simulink model "ss11"  (R2021b)
settings: Solver=ode23tb  StartTime=0.0  StopTime=25  FixedStep=1e-06  RelTol=1e-3  EnableMultiTasking=on
undefined symbols (not defined in the file): DiscIntNeverNeededParam, Par, sigbuilder_block, Ts
libraries: fl_lib x36, nesl_utility x30, ee_lib x12, simulink x9, simulink_extras x1, slpidlib x1
(part 1 of 2)
settings Model: SimulationMode=accelerator  Creator=Christo  LastModifiedBy=19840918
settings SolverCC: AlgebraicLoopSolver=TrustRegion  SolverResetMethod=Robust  AutoInsertRateTranBlk=on
settings DataIOCC: LimitDataPoints=on  SaveFormat=Array  ReturnWorkspaceOutputs=off
settings OptimizationCC: LifeSpan=inf
settings DebuggingCC: SolverPrmCheckMsg=warning  SFUnexpectedBacktrackingDiag=warning  SFNoUnconditionalDefaultTransitionDiag=warning  SFExecutionAtInitializationDiag=none  SFMachineParentedDataDiag=warning  ArithmeticOperatorsInVariantConditions=warning
settings HardwareCC: ProdBitPerPointer=32  ProdBitPerSizeT=32  ProdBitPerPtrDiffT=32  ProdLargestAtomicFloat=None  ProdIntDivRoundTo=Undefined  ProdEndianess=Unspecified  ProdWordSize=32  ProdHWDeviceType=32-bit Generic
settings ModelReferenceCC: PropagateSignalLabelsOutOfModel=off
settings SFSimCC: SimUseLocalCustomCode=off  CustomCodeUndefinedFunction=UseInterfaceOnly
settings RTWCC: RTWUseLocalCustomCode=off
settings CodeAppCC: StateflowObjectComments=on
settings GRTTargetCC: TargetLangStandard=C89/C90 (ANSI)
settings ConfigComp: CovMetricSettings=dw  CovSaveCumulativeToWorkspaceVar=on  CovSaveSingleToWorkspaceVar=on  CovExternalEMLEnable=off  CovSFcnEnable=off
settings SimscapeCC: SimscapeNormalizeSystem=off  SimscapeLogOpenViewer=on  SimscapeLogLimitData=off

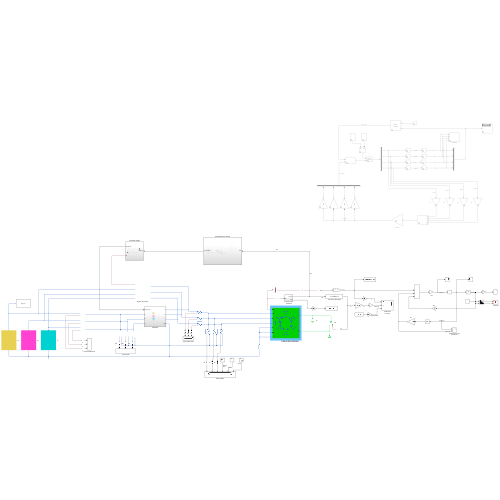
[thumbnail: Simulink's stored preview of the top-level diagram]
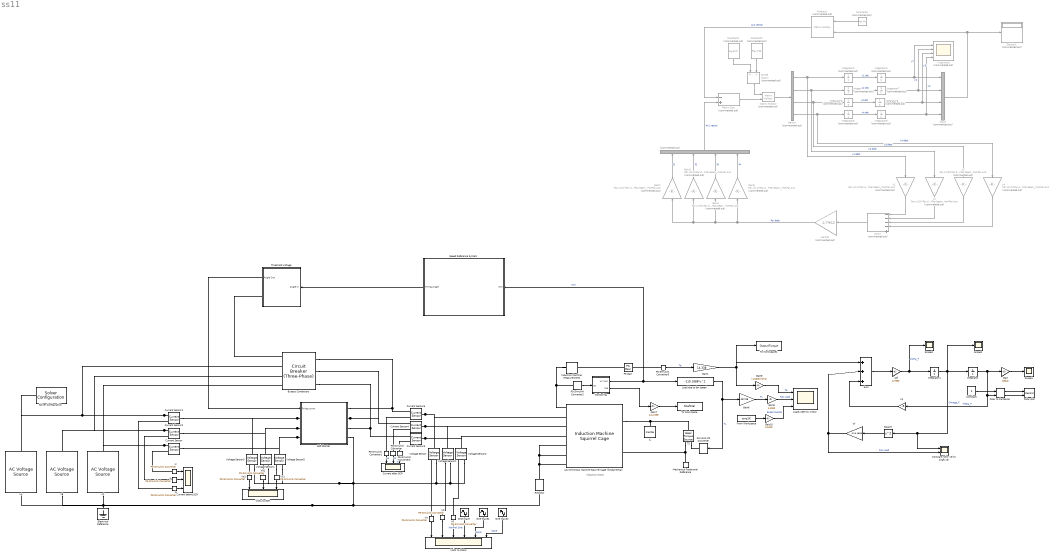
== system ss11 ==
  note: Induction Motor
  . : Mux  Commented=on
  1/Jf : Gain  Gain=1/7962
  Asynchronous Machine Squirrel Cage (fundamental) : ee_lib/Electromechanical/Asynchronous/Induction Machine Squirrel Cage  port_option=ee.enum.threePhasePort.expanded  SRated=250 kW  VRated=690 V  FRated=50 Hz  nPolePairs=2  param_unit=ee.enum.unit.si  squirrel_cage=ee.enum.squirrelcage.Single  zero_sequence=ee.enum.park.zerosequence.include  initialization_option=ee.enum.asm.initialization.fluxvariables  Rs=0.4 Ohm  Xls=0.5 Ohm  pu_Rs=0.0258  pu_Lls=0.0930  Rrd=0.04 Ohm  Xlrd=0.41/6 Ohm  pu_Rrd=0.0145  pu_Llrd=0.0424  Rrd1=0.28 Ohm  Xlrd1=0.82 Ohm  Rrd2=0.28 Ohm  Xlrd2=0.82 Ohm  pu_Rrd1=0.0290  pu_Llrd1=0.0848  pu_Rrd2=0.0290  pu_Llrd2=0.0848  Xm=17 Ohm  pu_Lm=1.7562  X0=0.9 Ohm  pu_L0=0.0930  saturation_option=ee.enum.saturation.exclude  saturation_i=[ 0,4,9,18,25,34,50,68,95,120 ] A  saturation_v=[ 0,88,154,198,220,242,264,286,308,330 ] V  pu_saturation_i=[0, .176, .396, .792, 1.1, 1.496, 2.2, 2.992, 4.18, 5.28]  pu_saturation_v=[0, .2309, .4041, .5196, .5774, .6351, .6928, .7506, .8083, .866]  connection_option=ee.enum.Connection.delta1  angular_position_specify=on  angular_position_priority=High  angular_position=0 deg  angular_position_nominal_specify=off  angular_position_nominal_unit=deg  angular_position_nominal_value=1  pu_psids_specify=off  pu_psids_priority=None  pu_psids=0  pu_psids_nominal_specify=off  pu_psids_nominal_unit=1  pu_psids_nominal_value=1  pu_psiqs_specify=off  pu_psiqs_priority=None  pu_psiqs=0  pu_psiqs_nominal_specify=off  pu_psiqs_nominal_unit=1  pu_psiqs_nominal_value=1  pu_psi0s_specify=off  pu_psi0s_priority=None  pu_psi0s=0  pu_psi0s_nominal_specify=off  pu_psi0s_nominal_unit=1  pu_psi0s_nominal_value=1  pu_psidr_specify=off  pu_psidr_priority=None  pu_psidr=0  pu_psidr_nominal_specify=off  pu_psidr_nominal_unit=1  pu_psidr_nominal_value=1  pu_psiqr_specify=off  pu_psiqr_priority=None  pu_psiqr=0  pu_psiqr_nominal_specify=off  pu_psiqr_nominal_unit=1  pu_psiqr_nominal_value=1  pu_psidr1_specify=off  pu_psidr1_priority=None  pu_psidr1=0  pu_psidr1_nominal_specify=off  pu_psidr1_nominal_unit=1  pu_psidr1_nominal_value=1  pu_psiqr1_specify=off  pu_psiqr1_priority=None  pu_psiqr1=0  pu_psiqr1_nominal_specify=off  pu_psiqr1_nominal_unit=1  pu_psiqr1_nominal_value=1  pu_psidr2_specify=off  pu_psidr2_priority=None  pu_psidr2=0  pu_psidr2_nominal_specify=off  pu_psidr2_nominal_unit=1  pu_psidr2_nominal_value=1  pu_psiqr2_specify=off  pu_psiqr2_priority=None  pu_psiqr2=0  pu_psiqr2_nominal_specify=off  pu_psiqr2_nominal_unit=1  pu_psiqr2_nominal_value=1  psids_specify=off  psids_priority=None  psids=0 Wb  psids_nominal_specify=off  psids_nominal_unit=Wb  psids_nominal_value=1  psiqs_specify=off  psiqs_priority=None  psiqs=0 Wb  psiqs_nominal_specify=off  psiqs_nominal_unit=Wb  psiqs_nominal_value=1  psi0s_specify=off  psi0s_priority=None  psi0s=0 Wb  psi0s_nominal_specify=off  psi0s_nominal_unit=Wb  psi0s_nominal_value=1  psidr_specify=off  psidr_priority=None  psidr=0 Wb  psidr_nominal_specify=off  psidr_nominal_unit=Wb  psidr_nominal_value=1  psiqr_specify=off  psiqr_priority=None  psiqr=0 Wb  psiqr_nominal_specify=off  psiqr_nominal_unit=Wb  psiqr_nominal_value=1  psidr1_specify=off  psidr1_priority=None  psidr1=0 Wb  psidr1_nominal_specify=off  psidr1_nominal_unit=Wb  psidr1_nominal_value=1  psiqr1_specify=off  psiqr1_priority=None  psiqr1=0 Wb  psiqr1_nominal_specify=off  psiqr1_nominal_unit=Wb  psiqr1_nominal_value=1  psidr2_specify=off  psidr2_priority=None  psidr2=0 Wb  psidr2_nominal_specify=off  psidr2_nominal_unit=Wb  psidr2_nominal_value=1  psiqr2_specify=off  psiqr2_priority=None  psiqr2=0 Wb  psiqr2_nominal_specify=off  psiqr2_nominal_unit=Wb  psiqr2_nominal_value=1  slip_specify=off  slip_priority=None  slip=0  slip_nominal_specify=off  slip_nominal_unit=1  slip_nominal_value=1  real_power_generated_specify=off  real_power_generated_priority=None  real_power_generated=0 W  real_power_generated_nominal_specify=off  real_power_generated_nominal_unit=W  real_power_generated_nominal_value=1  mechanical_power_consumed_specify=off  mechanical_power_consumed_priority=None  mechanical_power_consumed=0 W  mechanical_power_consumed_nominal_specify=off  mechanical_power_consumed_nominal_unit=W  mechanical_power_consumed_nominal_value=1  Tmeas=298.15 K  alpha=3.93e-3 1/K  alpha_cage=4.4e-3 1/K  stator_thermal_mass=100 J/K  rotor_thermal_mass=200 J/K  temperatureA_specify=off  temperatureA_priority=High  temperatureA=25 degC  temperatureA_nominal_specify=off  temperatureA_nominal_unit=degC  temperatureA_nominal_value=1  temperatureB_specify=off  temperatureB_priority=High  temperatureB=25 degC  temperatureB_nominal_specify=off  temperatureB_nominal_unit=degC  temperatureB_nominal_value=1  temperatureC_specify=off  temperatureC_priority=High  temperatureC=25 degC  temperatureC_nominal_specify=off  temperatureC_nominal_unit=degC  temperatureC_nominal_value=1  temperatureR_specify=off  temperatureR_priority=High  temperatureR=25 degC  temperatureR_nominal_specify=off  temperatureR_nominal_unit=degC  temperatureR_nominal_value=1
      settings: SourceProductBaseCode=PS  InternalSimscapePortConfiguration="{\"Bottom\":[],\"Left\":[{\"id\":\"R\",\"label\":\"R\",\"type\":\"foundation.mechanical.rotational.rotational\"},{\"id\":\"C\",\"label\":\"C\",\"type\":\"foundation.mechanical.rotational.rotational\"}],\"Right\":[{\"id\":\"pu_output\",\"label\":\"pu\",\"type\":\"output\"},{\"id\":\"a1\",\"label\":\"a1\",\"type\":\"foundation.electrical.electrical\"},{\"id\":\"b1\",\"label\":\"b1\",\"type\":\"foundation.electrical.electrical\"},{\"id\":\"c1\",\"label\":\"c1\",\"type\":\"foundation.electrical.electrical\"},{\"id\":\"a2\",\"label\":\"a2\",\"type\":\"foundation.electrical.electrical\"},{\"id\":\"b2\",\"label\":\"b2\",\"type\":\"foundation.electrical.electrical\"},{\"id\":\"c2\",\"label\":\"c2\",\"type\":\"foundation.electrical.electrical\"}],\"Top\":[]}"
  Bypass Contactors : ee_lib/Switches & Breakers/Circuit Breaker (Three-Phase)  R_closed=0.0001 Ohm  G_open=1e-6 1/Ohm  threshold=2 V
      settings: SourceProductBaseCode=PS  LogSimulationData=on  InternalSimscapePortConfiguration="{\"Bottom\":[],\"Left\":[{\"id\":\"vT\",\"label\":\"vT\",\"type\":\"input\"},{\"id\":\"a1\",\"label\":\"a1\",\"type\":\"foundation.electrical.electrical\"},{\"id\":\"b1\",\"label\":\"b1\",\"type\":\"foundation.electrical.electrical\"},{\"id\":\"c1\",\"label\":\"c1\",\"type\":\"foundation.electrical.electrical\"}],\"Right\":[{\"id\":\"a2\",\"label\":\"a2\",\"type\":\"foundation.electrical.electrical\"},{\"id\":\"b2\",\"label\":\"b2\",\"type\":\"foundation.electrical.electrical\"},{\"id\":\"c2\",\"label\":\"c2\",\"type\":\"foundation.electrical.electrical\"}],\"Top\":[]}"
  Compare rotor vel to shaft vel : Scope  NumInputPorts=2
  Constant : Constant
  Constant1 : Constant  Commented=on  Value=eye(4)
  Constant2 : Constant  Commented=on  Value=Par.Mb
  Constant3 : Constant  Commented=on  Value=Par.Kb
  Current Sensor{,1..5} (6 alike) : fl_lib/Electrical/Electrical Sensors/Current Sensor
  Current after SCR : Scope  NumInputPorts=3
  Current before SCR : Scope  NumInputPorts=3
  Demux : Demux  Commented=on
  Display1 : Display  Commented=on
  Divide : Product  Commented=on  Inputs=*/  Multiplication=Matrix(*)
  Electrical Reference : fl_lib/Electrical/Electrical Elements/Electrical Reference
  From Workspace : FromWorkspace  VariableName=torq1K
  Gain : Gain  Gain=180/pi
  Gain1 : Gain  Gain=14.338
  Gain10 : Gain  Gain=1/1000
  Gain2 : Gain  Commented=on  Gain=Par.xc(1)*Par.delta_x*Par.beam_rho*Par.Acs
  Gain3 : Gain  Commented=on  Gain=Par.xc(2)*Par.delta_x*Par.beam_rho*Par.Acs
  Gain4 : Gain  Commented=on  Gain=Par.xc(3)*Par.delta_x*Par.beam_rho*Par.Acs
  Gain5 : Gain  Commented=on  Gain=Par.xc(4)*Par.delta_x*Par.beam_rho*Par.Acs
  Gain6 : Gain  Gain=-157.08
  Gain7 : Gain  Gain=1/14.338
  Gain8 : Gain  Gain=(1/1000)*2*pi
  Gain9 : Gain  Gain=1/1000
  Ia : nesl_utility/PS-Simulink Converter  PhysicalDomain=network_engine_domain  SubClassName=ps_output  LeftPortType=input  RightPortType=output  PseudoPeriodic=off  Frequencies=[]  Unit=A  AffineConversion=off
      settings: SourceProductBaseCode=PW,SS
  Ib : nesl_utility/PS-Simulink Converter  PhysicalDomain=network_engine_domain  SubClassName=ps_output  LeftPortType=input  RightPortType=output  PseudoPeriodic=off  Frequencies=[]  Unit=A  AffineConversion=off
      settings: SourceProductBaseCode=PW,SS
  Ic : nesl_utility/PS-Simulink Converter  PhysicalDomain=network_engine_domain  SubClassName=ps_output  LeftPortType=input  RightPortType=output  PseudoPeriodic=off  Frequencies=[]  Unit=A  AffineConversion=off
      settings: SourceProductBaseCode=PW,SS
  Induction Machine Measurement1 : ee_lib/Electromechanical/Asynchronous/Induction Machine Measurement  output_idx=1
      settings: SourceProductBaseCode=PS  InternalSimscapePortConfiguration="{\"Bottom\":[],\"Left\":[{\"id\":\"pu_input\",\"label\":\"pu\",\"type\":\"input\"}],\"Right\":[{\"id\":\"pu_output\",\"label\":\"o\",\"type\":\"output\"}],\"Top\":[]}"
  Inertias : Gain  Commented=on  Gain=1/7962
  Integrator : Integrator
  Integrator1 : Integrator
  Integrator{2..9} (8 alike) : Integrator  Commented=on
  JL : fl_lib/Mechanical/Rotational Elements/Inertia  inertia=6.3+10+7962/(14.32^2) kg*m^2  num_ports=foundation.enum.numPorts2.one  w_specify=off  w_priority=High  w=0 rad/s  w_nominal_specify=off  w_nominal_unit=rad/s  w_nominal_value=1  t_specify=off  t_priority=High  t=0 N*m  t_nominal_specify=off  t_nominal_unit=N*m  t_nominal_value=1
  Kf : Gain  Gain=-119.1888
  Ks : Gain  Gain=-5
  Load due to fan speed : Fcn  Expr=-119.1888*u^2
  Loads seen by motor : Scope  NumInputPorts=3
  Matrix Sum : Sum  Commented=on  Inputs=-+
  Matrix Multiply : Product  Commented=on  Multiplication=Matrix(*)
  Mechanical Rotational Reference : fl_lib/Mechanical/Rotational Elements/Mechanical Rotational Reference
  Monitoring : Subsystem
  Mux2 : Mux  Commented=on
  PS Gain : fl_lib/Physical Signals/Functions/PS Gain  gain=1591.55 N*m
  PS-Simulink Converter{,1,3,5} (4 alike) : nesl_utility/PS-Simulink Converter  PhysicalDomain=network_engine_domain  SubClassName=ps_output  LeftPortType=input  RightPortType=output  PseudoPeriodic=off  Frequencies=[]  Unit=inherit  AffineConversion=off
      settings: SourceProductBaseCode=PW,SS
  PS-Simulink Converter2 : nesl_utility/PS-Simulink Converter  PhysicalDomain=network_engine_domain  SubClassName=ps_output  LeftPortType=input  RightPortType=output  PseudoPeriodic=off  Frequencies=[]  Unit=1  AffineConversion=off
      settings: SourceProductBaseCode=PW,SS
  Polar plot : Record  FileSettingsInternal="{\"entries\":[{\"content\":{\"excelSettings\":{\"content\":{},\"type\":\"Streamout.ExcelSettings\"}},\"type\":\"Streamout.FileSettingStorage\",\"uuid\":\"54fc2ee3-5b5e-4f8c-8741-d132ad52efdf\"}],\"packageUris\":[\"http://schema.mathworks.com/mf0/streamout_blocks/R2020a\"],\"version\":\"1.0\"}"  Layout=[1 1]  SignalsInternal="{\"entries\":[{\"content\":{\"signals\":[{\"content\":{\"blockPath\":[\"ss11/Polar plot\"],\"channel\":[],\"dimensions\":[1],\"domain\":\"ss11/Polar plot\",\"lineColor\":\"#77ac30\",\"plots\":[],\"port\":1,\"sid\":[\"\"],\"signalID\":639,\"signalName\":\"Polar to\\nCartesian:1\"},\"type\":\"RecordBlkView.Signal\",\"uuid\":\"d88677cd-d414-4038-8e24-bb5f350f4e87\"},{\"content\":{\"blockPath\":[\"ss11/Polar plot\"],\"channel\":[],\"dimensions\":[1],\"domain\":\"ss11/Polar plot\",\"lineColor\":\"#4dbeee\",\"plots\":[],\"port\":2,\"sid\":[\"\"],\"signalID\":643,\"signalName\":\"Polar to\\nCartesian:2\"},\"type\":\"RecordBlkView.Signal\",\"uuid\":\"c3000e72-a674-483a-a6e8-47c6664286a5\"}]},\"type\":\"RecordBlkView.InputSignals\",\"uuid\":\"32de7f82-7389-4a3b-8503-0a628280bb19\"}],\"packageUris\":[\"http://schema.mathworks.com/mf0/streamout_blocks/R2020a\"],\"version\":\"1.0\"}"  VisualizationBindings="{\"xyplotplugin\":{\"info\":[{\"series\":[],\"subplotID\":1}]}}"  CompatibilityTag=XY
  Polar to Cartesian : simulink_extras/Transformations/Polar to Cartesian
      settings: SourceProductBaseCode=SL
  Product1 : Product  Commented=on  Multiplication=Matrix(*)
  Resistor : fl_lib/Electrical/Electrical Elements/Resistor  R=1e09 Ohm  i_specify=off  i_priority=None  i=0 A  i_nominal_specify=off  i_nominal_unit=A  i_nominal_value=1  v_specify=off  v_priority=None  v=0 V  v_nominal_specify=off  v_nominal_unit=V  v_nominal_value=1
  Scope1 : Scope
  Scope2 : Scope
  Scope3 : Scope
  Simulink-PS Converter : nesl_utility/Simulink-PS Converter  PhysicalDomain=network_engine_domain  SubClassName=ps_input  LeftPortType=input  RightPortType=output  PseudoPeriodic=off  Frequencies=[]  NoiseDistribution=none  NoiseParameters=[]  Unit=N*m  AffineConversion=off  FilteringAndDerivatives=zero  SimscapeFilterOrder=1  InputFilterTimeConstant=0.001  UdotUserProvided=1
      settings: SourceProductBaseCode=PW,SS
  Sine Wave : Sin  Amplitude=690  Frequency=2*pi*50  SampleTime=0
  Sine Wave1 : Sin  Amplitude=690  Frequency=2*pi*50  Phase=2*pi/3  SampleTime=0
  Sine Wave2 : Sin  Amplitude=690  Frequency=2*pi*50  Phase=-2*pi/3  SampleTime=0
  Soft Starter : Subsystem
  Solver Configuration : nesl_utility/Solver Configuration  PhysicalDomain=network_engine_domain  SubClassName=solver  LeftPortType=input  RightPortType=generic  Tones=[]  Harmonics=[]  SimulateNoise=off  Profile=off  UseLocalSampling=off  EnableSwitchedLinearOptims=on  FrequencyDomain=off  UseCCode=off  RelTol=0.001  AbsTol=1e-06  MinStep=1e-09  ToWorkspace=off  RevertToSquareIcSolve=off  NumHomotopyIterations=100  PhasorMode=off  PhasorModeNumHarmonics=1  DoDC=off  ResidualTolerance=1e-09  UseLocalSolver=on  LocalSolverChoice=NE_BACKWARD_EULER_ADVANCER  LocalSolverSampleTime=1.0e-04  DoFixedCost=on  MaxNonlinIter=3  MaxModeIter=2  ComputeImpulses=off  ImpulseIterations=2  LinearAlgebra=Sparse  EquationFormulation=NE_TIME_EF  DelaysMemoryBudget=1024  AutomaticFiltering=on  FilteringTimeConstant=0.001  PartitionStorageMethod=AS_NEEDED  PartitionMemoryBudget=1024  PartitionMethod=FAST
      settings: SourceProductBaseCode=PW,SS
  Speed Reference System : Subsystem
  Square : Math  Operator=square  SaturateOnIntegerOverflow=on
  Sum : Sum  Inputs=|+++
  Sum2 : Sum  Commented=on  Inputs=----+
  TS : fl_lib/Mechanical/Mechanical Sources/Ideal Torque Source
  Threshold Voltage : Subsystem
  To Workspace : ToWorkspace  VariableName=ShaftVel  SaveFormat=Timeseries  SampleTime=-1
  To Workspace1 : ToWorkspace  VariableName=OutputTorque  SaveFormat=Timeseries  SampleTime=-1
  Va : nesl_utility/PS-Simulink Converter  PhysicalDomain=network_engine_domain  SubClassName=ps_output  LeftPortType=input  RightPortType=output  PseudoPeriodic=off  Frequencies=[]  Unit=inherit  AffineConversion=off
      settings: SourceProductBaseCode=PW,SS
  Va1 : nesl_utility/PS-Simulink Converter  PhysicalDomain=network_engine_domain  SubClassName=ps_output  LeftPortType=input  RightPortType=output  PseudoPeriodic=off  Frequencies=[]  Unit=inherit  AffineConversion=off
      settings: SourceProductBaseCode=PW,SS
  Vb : nesl_utility/PS-Simulink Converter  PhysicalDomain=network_engine_domain  SubClassName=ps_output  LeftPortType=input  RightPortType=output  PseudoPeriodic=off  Frequencies=[]  Unit=inherit  AffineConversion=off
      settings: SourceProductBaseCode=PW,SS
  Vb1 : nesl_utility/PS-Simulink Converter  PhysicalDomain=network_engine_domain  SubClassName=ps_output  LeftPortType=input  RightPortType=output  PseudoPeriodic=off  Frequencies=[]  Unit=inherit  AffineConversion=off
      settings: SourceProductBaseCode=PW,SS
  Vc : nesl_utility/PS-Simulink Converter  PhysicalDomain=network_engine_domain  SubClassName=ps_output  LeftPortType=input  RightPortType=output  PseudoPeriodic=off  Frequencies=[]  Unit=inherit  AffineConversion=off
      settings: SourceProductBaseCode=PW,SS
  Vc1 : nesl_utility/PS-Simulink Converter  PhysicalDomain=network_engine_domain  SubClassName=ps_output  LeftPortType=input  RightPortType=output  PseudoPeriodic=off  Frequencies=[]  Unit=inherit  AffineConversion=off
      settings: SourceProductBaseCode=PW,SS
  Voltage Sensor{,1..5} (6 alike) : fl_lib/Electrical/Electrical Sensors/Voltage Sensor
  Volts to Motor : Scope  NumInputPorts=6
  Volts to SCR : Scope  NumInputPorts=3
  Y-positions : Scope  Commented=on  NumInputPorts=4
  vA : fl_lib/Electrical/Electrical Sources/AC Voltage Source  amp=690 V  shift=0 deg  frequency=50 Hz  omega=0 rad/s
  vB : fl_lib/Electrical/Electrical Sources/AC Voltage Source  amp=690 V  shift=-120 deg  frequency=50 Hz  omega=0 rad/s
  vC : fl_lib/Electrical/Electrical Sources/AC Voltage Source  amp=690 V  shift=120 deg  frequency=50 Hz  omega=0 rad/s
  y1 : Gain  Commented=on  Gain=Par.xc(1)*Par.delta_x*Par.beam_rho*Par.Acs
  y2 : Gain  Commented=on  Gain=Par.xc(2)*Par.delta_x*Par.beam_rho*Par.Acs
  y3 : Gain  Commented=on  Gain=Par.xc(3)*Par.delta_x*Par.beam_rho*Par.Acs
  y4 : Gain  Commented=on  Gain=Par.xc(4)*Par.delta_x*Par.beam_rho*Par.Acs
  wires:
  PS-Simulink Converter2/1 -> Monitoring/1(pu)
  PS-Simulink Converter5/1 -> Gain1/1  "Te"
  Vb/1 -> Volts to Motor/2
  PS-Simulink Converter1/1 -> Current after SCR/1  "Ia"
  PS-Simulink Converter3/1 -> Current after SCR/3  "Ic"
  PS-Simulink Converter/1 -> Current after SCR/2  "Ib"
  Ia/1 -> Current before SCR/3
  Ib/1 -> Current before SCR/2
  1/Jf/1 -> Integrator1/1, Scope3/1  "Alpha_F"
  Gain/1 -> Scope1/1
  Polar to Cartesian/2 -> Polar plot/2
  Constant/1 -> Polar to Cartesian/1
  Polar to Cartesian/1 -> Polar plot/1
  Speed Reference System/1(Firing Angle) -> Threshold Voltage/1(Angle In)
  Threshold Voltage/1(Angle Out) -> Soft Starter/1(firing curve)
  Monitoring/1(wr (pu)) -> Load due to fan speed/1, Speed Reference System/1(Win)  "Win"
  Ic/1 -> Current before SCR/1
  Sine Wave2/1 -> Volts to Motor/6  "-2pi/3"
  Sine Wave/1 -> Volts to Motor/4  "Normal Sine"
  Integrator/1 -> Gain/1, Ks/1, Polar to Cartesian/2  "Theta_F"
  Va1/1 -> Volts to SCR/1
  Va/1 -> Volts to Motor/1
  Kf/1 -> Compare rotor vel to shaft vel/2, Sum/2  "Fan Load"
  Sine Wave1/1 -> Volts to Motor/5  "2pi/3"
  Square/1 -> Kf/1
  Integrator1/1 -> Integrator/1, Scope2/1, Compare rotor vel to shaft vel/1, Square/1  "Omega_F"
  Vc/1 -> Volts to Motor/3
  Sum/1 -> 1/Jf/1
  Vc1/1 -> Volts to SCR/3
  Vb1/1 -> Volts to SCR/2
  y4/1 -> Sum2/4
  Demux/3 -> Integrator5/1, y3/1  "y3 ddot"
  Gain2/1 -> ./1  "f1"
  Integrator3/1 -> Y-positions/1, Mux2/1  "y1"
  y3/1 -> Sum2/3
  Integrator4/1 -> Integrator7/1  "y2 dot"
  Demux/1 -> Integrator2/1, y1/1  "y1 ddot"
  Integrator9/1 -> Y-positions/4, Mux2/4  "y4"
  Gain3/1 -> ./2  "f2"
  Constant3/1 -> Product1/1
  Integrator8/1 -> Y-positions/3, Mux2/3  "y3"
  Inertias/1 -> Gain2/1, Gain3/1, Gain4/1, Gain5/1  "Psi ddot"
  y1/1 -> Sum2/1
  Matrix Multiply/1 -> Demux/1
  Constant1/1 -> Divide/1
  Integrator5/1 -> Integrator8/1  "y3 dot"
  Gain5/1 -> ./4  "f4"
  Gain4/1 -> ./3  "f3"
  Demux/4 -> Integrator6/1, y4/1  "y4 ddot"
  Integrator7/1 -> Y-positions/2, Mux2/2  "y2"
  Sum2/1 -> Inertias/1
  y2/1 -> Sum2/2
  Demux/2 -> Integrator4/1, y2/1  "y2 ddot"
  Divide/1 -> Matrix Multiply/1
  Product1/1 -> Matrix Sum/1  "4x1 vector"
  Integrator2/1 -> Integrator3/1  "y1 dot"
  Matrix Sum/1 -> Matrix Multiply/2
  Constant2/1 -> Divide/2
  Integrator6/1 -> Integrator9/1  "y4 dot"
  Mux2/1 -> Product1/2, Display1/1
  ./1 -> Matrix Sum/2  "4x1 vector"
  Load due to fan speed/1 -> Simulink-PS Converter/1, Gain6/1  "TL"
  Gain1/1 -> Sum/1, To Workspace1/1, Gain8/1
  Ks/1 -> Sum/3
  Gain7/1 -> To Workspace/1
  Monitoring/2(We) -> Gain7/1
  Gain6/1 -> Gain9/1  "TL"
  Gain9/1 -> Loads seen by motor/2  "Fan Load"
  Gain10/1 -> Loads seen by motor/3  "Experimental"
  From Workspace/1 -> Gain10/1
  Gain8/1 -> Loads seen by motor/1  "Te"
  connections:
  Current Sensor4/LConn1 -- Asynchronous Machine Squirrel Cage (fundamental)/RConn3 -- Voltage Sensor1/LConn1
  Soft Starter/RConn2 -- Current Sensor4/RConn2 -- Bypass Contactors/RConn2
  Current Sensor1/RConn2 -- Bypass Contactors/LConn2 -- vA/LConn1 -- Solver Configuration/RConn1
  Soft Starter/LConn3 -- Current Sensor/LConn1 -- Voltage Sensor5/LConn1
  Current Sensor5/LConn1 -- Asynchronous Machine Squirrel Cage (fundamental)/RConn2 -- Voltage Sensor/LConn1
  TS/RConn2 -- Asynchronous Machine Squirrel Cage (fundamental)/LConn2 -- Mechanical Rotational Reference/LConn1
  Asynchronous Machine Squirrel Cage (fundamental)/RConn7 -- Asynchronous Machine Squirrel Cage (fundamental)/RConn5 -- Asynchronous Machine Squirrel Cage (fundamental)/RConn6 -- Resistor/LConn1
  Soft Starter/LConn2 -- Current Sensor2/LConn1 -- Voltage Sensor4/LConn1
  Bypass Contactors/RConn1 -- Soft Starter/RConn1 -- Current Sensor5/RConn2
  JL/LConn1 -- TS/LConn1 -- Asynchronous Machine Squirrel Cage (fundamental)/LConn1
  Bypass Contactors/RConn3 -- Soft Starter/RConn3 -- Current Sensor3/RConn2
  Current Sensor3/LConn1 -- Asynchronous Machine Squirrel Cage (fundamental)/RConn4 -- Voltage Sensor2/LConn1
  Voltage Sensor2/RConn2 -- Voltage Sensor3/RConn2 -- Voltage Sensor4/RConn2 -- Voltage Sensor5/RConn2 -- Soft Starter/RConn4 -- Resistor/RConn1 -- Electrical Reference/LConn1 -- vC/RConn1 -- vA/RConn1 -- vB/RConn1 -- Voltage Sensor/RConn2 -- Voltage Sensor1/RConn2
  Current Sensor2/RConn2 -- vB/LConn1 -- Bypass Contactors/LConn3
  Induction Machine Measurement1/LConn1 -- PS-Simulink Converter2/LConn1 -- Asynchronous Machine Squirrel Cage (fundamental)/RConn1
  Current Sensor/RConn2 -- vC/LConn1 -- Bypass Contactors/LConn4
  Soft Starter/LConn1 -- Current Sensor1/LConn1 -- Voltage Sensor3/LConn1
  Current Sensor3/RConn1 -- PS-Simulink Converter3/LConn1
  Voltage Sensor4/RConn1 -- Vb1/LConn1
  Current Sensor1/RConn1 -- Ia/LConn1
  Va1/LConn1 -- Voltage Sensor3/RConn1
  PS-Simulink Converter1/LConn1 -- Current Sensor5/RConn1
  PS Gain/LConn1 -- Induction Machine Measurement1/RConn1
  Threshold Voltage/RConn1 -- Bypass Contactors/LConn1
  Va/LConn1 -- Voltage Sensor/RConn1
  Current Sensor4/RConn1 -- PS-Simulink Converter/LConn1
  Vc/LConn1 -- Voltage Sensor2/RConn1
  Voltage Sensor5/RConn1 -- Vc1/LConn1
  Voltage Sensor1/RConn1 -- Vb/LConn1
  Current Sensor2/RConn1 -- Ib/LConn1
  Ic/LConn1 -- Current Sensor/RConn1
  PS-Simulink Converter5/LConn1 -- PS Gain/RConn1
  TS/RConn1 -- Simulink-PS Converter/RConn1

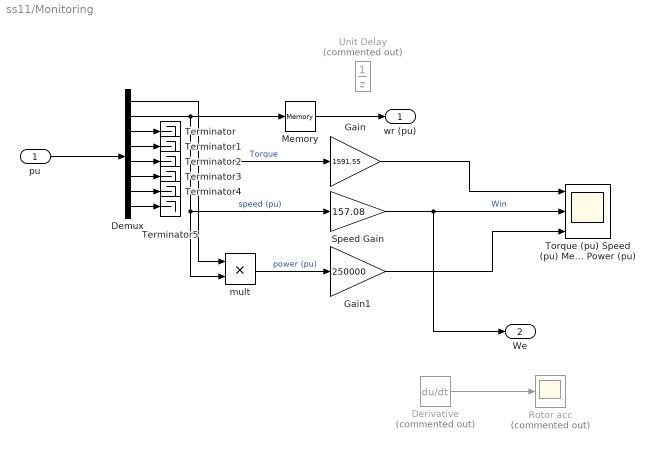
== system ss11/Monitoring ==
  pu : Inport
  Demux : Demux  Outputs=8
  Derivative : Derivative  Commented=on
  Gain : Gain  Gain=1591.55
  Gain1 : Gain  Gain=250000
  Memory : Memory
  Rotor acc : Scope  Commented=on
  Speed Gain : Gain  Gain=157.08
  Terminator{,1..5} (6 alike) : Terminator
  "Torque (pu) Speed (pu) Mech Power (pu) " : Scope  NumInputPorts=3
  Unit Delay : UnitDelay  Commented=on  SampleTime=-1  HasFrameUpgradeWarning=on
  mult : Product  Inputs=**
  wr (pu) : Outport
  We : Outport  Port=2
  wires:
  pu/1 -> Demux/1
  Demux/2 -> Memory/1, mult/2, Speed Gain/1  "speed (pu)"
  mult/1 -> Gain1/1  "power (pu)"
  Demux/1 -> mult/1, Gain/1  "Torque"
  Demux/3 -> Terminator/1
  Demux/8 -> Terminator5/1
  Demux/7 -> Terminator4/1
  Demux/6 -> Terminator3/1
  Demux/5 -> Terminator2/1
  Demux/4 -> Terminator1/1
  Gain1/1 -> "Torque (pu) Speed (pu) Mech Power (pu) "/3
  Derivative/1 -> Rotor acc/1
  Speed Gain/1 -> We/1, "Torque (pu) Speed (pu) Mech Power (pu) "/2  "Win"
  Gain/1 -> "Torque (pu) Speed (pu) Mech Power (pu) "/1
  Memory/1 -> wr (pu)/1

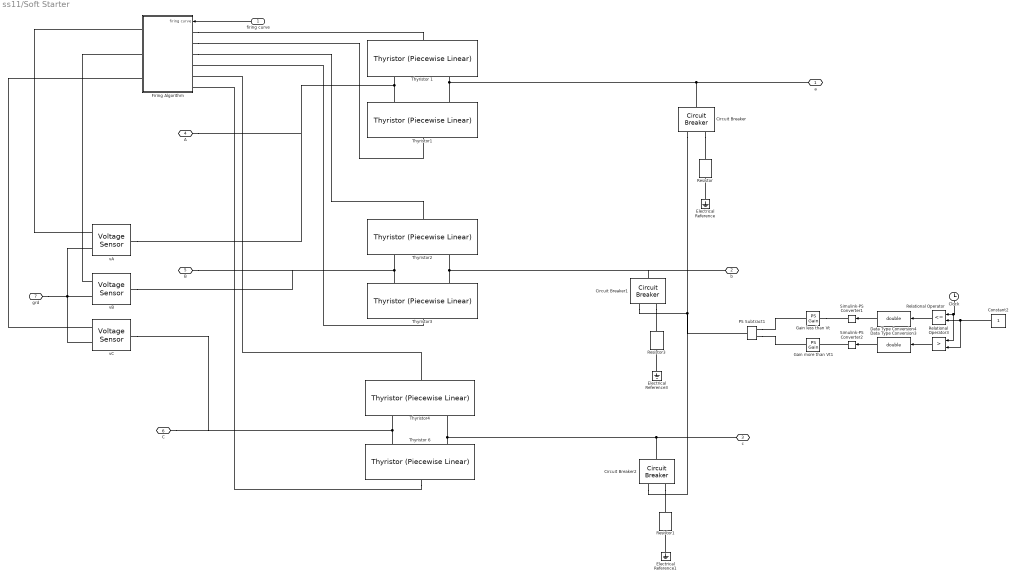
== system ss11/Soft Starter ==
  firing curve : Inport
  Circuit Breaker : ee_lib/Switches & Breakers/Circuit Breaker  R_closed=0.001 Ohm  G_open=1e-6 1/Ohm  threshold=2 V  offset_for_on=1 V
      settings: SourceProductBaseCode=PS  InternalSimscapePortConfiguration="{\"Bottom\":[],\"Left\":[{\"id\":\"vT\",\"label\":\"vT\",\"type\":\"input\"},{\"id\":\"p1\",\"label\":\"\",\"type\":\"foundation.electrical.electrical\"}],\"Right\":[{\"id\":\"p2\",\"label\":\"\",\"type\":\"foundation.electrical.electrical\"}],\"Top\":[]}"
  Circuit Breaker1 : ee_lib/Switches & Breakers/Circuit Breaker  R_closed=0.001 Ohm  G_open=1e-6 1/Ohm  threshold=2 V  offset_for_on=1 V
      settings: SourceProductBaseCode=PS  InternalSimscapePortConfiguration="{\"Bottom\":[],\"Left\":[{\"id\":\"vT\",\"label\":\"vT\",\"type\":\"input\"},{\"id\":\"p1\",\"label\":\"\",\"type\":\"foundation.electrical.electrical\"}],\"Right\":[{\"id\":\"p2\",\"label\":\"\",\"type\":\"foundation.electrical.electrical\"}],\"Top\":[]}"
  Circuit Breaker2 : ee_lib/Switches & Breakers/Circuit Breaker  R_closed=0.001 Ohm  G_open=1e-6 1/Ohm  threshold=2 V  offset_for_on=1 V
      settings: SourceProductBaseCode=PS  InternalSimscapePortConfiguration="{\"Bottom\":[],\"Left\":[{\"id\":\"vT\",\"label\":\"vT\",\"type\":\"input\"},{\"id\":\"p1\",\"label\":\"\",\"type\":\"foundation.electrical.electrical\"}],\"Right\":[{\"id\":\"p2\",\"label\":\"\",\"type\":\"foundation.electrical.electrical\"}],\"Top\":[]}"
  Clock : Clock
  Constant2 : Constant
  Data Type Conversion3 : DataTypeConversion  OutDataTypeStr=double
  Data Type Conversion4 : DataTypeConversion  OutDataTypeStr=double
  Electrical Reference : fl_lib/Electrical/Electrical Elements/Electrical Reference
  Electrical Reference1 : fl_lib/Electrical/Electrical Elements/Electrical Reference
  Electrical Reference3 : fl_lib/Electrical/Electrical Elements/Electrical Reference
  Firing Algorithm : Subsystem
  Gain less than Vt : fl_lib/Physical Signals/Functions/PS Gain  gain=-1 V
  Gain more than Vt1 : fl_lib/Physical Signals/Functions/PS Gain  gain=3 V
  PS Subtract1 : fl_lib/Physical Signals/Functions/PS Subtract
  Relational Operator : RelationalOperator  Operator=<=  OutDataTypeStr=boolean  RndMeth=Simplest
  Relational Operator3 : RelationalOperator  Operator=>  OutDataTypeStr=boolean  RndMeth=Simplest
  Resistor : fl_lib/Electrical/Electrical Elements/Resistor  R=0.01 Ohm  i_specify=off  i_priority=None  i=0 A  i_nominal_specify=off  i_nominal_unit=A  i_nominal_value=1  v_specify=off  v_priority=None  v=0 V  v_nominal_specify=off  v_nominal_unit=V  v_nominal_value=1
  Resistor1 : fl_lib/Electrical/Electrical Elements/Resistor  R=0.01 Ohm  i_specify=off  i_priority=None  i=0 A  i_nominal_specify=off  i_nominal_unit=A  i_nominal_value=1  v_specify=off  v_priority=None  v=0 V  v_nominal_specify=off  v_nominal_unit=V  v_nominal_value=1
  Resistor3 : fl_lib/Electrical/Electrical Elements/Resistor  R=0.01 Ohm  i_specify=off  i_priority=None  i=0 A  i_nominal_specify=off  i_nominal_unit=A  i_nominal_value=1  v_specify=off  v_priority=None  v=0 V  v_nominal_specify=off  v_nominal_unit=V  v_nominal_value=1
  Simulink-PS Converter1 : nesl_utility/Simulink-PS Converter  PhysicalDomain=network_engine_domain  SubClassName=ps_input  LeftPortType=input  RightPortType=output  PseudoPeriodic=off  Frequencies=[]  NoiseDistribution=none  NoiseParameters=[]  Unit=1  AffineConversion=off  FilteringAndDerivatives=provide  SimscapeFilterOrder=1  InputFilterTimeConstant=0.001  UdotUserProvided=0
      settings: SourceProductBaseCode=PW,SS
  Simulink-PS Converter2 : nesl_utility/Simulink-PS Converter  PhysicalDomain=network_engine_domain  SubClassName=ps_input  LeftPortType=input  RightPortType=output  PseudoPeriodic=off  Frequencies=[]  NoiseDistribution=none  NoiseParameters=[]  Unit=1  AffineConversion=off  FilteringAndDerivatives=provide  SimscapeFilterOrder=1  InputFilterTimeConstant=0.001  UdotUserProvided=0
      settings: SourceProductBaseCode=PW,SS
  Thyristor 1 : ee_lib/Semiconductors & Converters/Thyristor (Piecewise Linear)  Vf=0.8 V  Ron=0.001 Ohm  Goff=1.0000e-05 1/Ohm  Vgt=6 V  Ih=0.01 A  diode_param=1  diode_Vf=0.8 V  diode_Ron=0.001 Ohm  diode_Goff=1e-5 1/Ohm  diode_C=5e-8 F  diode_iRM=-235 A  diode_iF=300 A  diode_idot=-50 A/us  diode_trr_param=1  diode_trr_factor=3  diode_trr=15 us  diode_Qrr=1.5e+3 s*uA  thermal_loss_option=ee.enum.converters.thermalLossOption.constantvalues  Von_data=[0, .1, .6, .8, 1, 1.3, 1.6, 2, 2.4; 0, .1, .7, 1, 1.2, 1.5, 1.9, 2.4, 2.8] V  Tj=[298.15, 398.15] K  Iout_data=[0, .1, 1, 5, 10, 20, 40, 70, 100] A  Eon_data=[0, .0024, .024, .12, .2, .48, 1.04, 2.16, 3.24; 0, .003, .03, .15, .25, .6, 1.3, 2.7, 4.05] * 1e-3 J  Tj_loss=[298.15, 398.15] K  Iout_data_loss=[0, .1, 1, 5, 10, 20, 40, 70, 100] A  Eon_scalar=22.86e-3 J  Eoff_natural_commutation=10e-3 J  Voff=300 V  Iout_scalar=600 A  onCurrentMeasDelay=1e-4 s  diodeModelType=ee.enum.converters.diodeModelType.pwl  diodeTableType=ee.enum.diode.tableType.IfMat  diode_IfMat=[.07, .12, .19, 1.75, 4.24, 7.32, 11.2; .16, .3, .72, 2.14, 4.02, 6.35, 9.12] A  diode_VfMat=[.9, 1.15, 1.25, 1.5, 1.75, 2.17, 2.6, 2.85; .58, .68, .75, 1.1, 1.38, 1.77, 2.27, 2.7] V  diode_TjVec=[25, 125] degC  diode_VfVec=[.5, .7, .9, 1.3, 1.7, 2.1, 2.5] V  diode_IfVec=[.1, .2, .5, 1, 2, 4, 7, 10] A  thermal_network_parameterization=ee.enum.thermalNetworkTopology.external  Rth=[.08, .5] K/W  Rth_Cauer=[.08, .1, .5] K/W  Rth_Foster=[.08, .14, .22, .16] K/W  thermal_mass_parameterization=ee.enum.thermalNetwork.timeconstant  thermal_mass=[.01, .5] J/K  thermal_mass_Cauer=[.01, .1, .5] J/K  thermal_mass_Foster=[.001, .005, .05, .5] J/K  thermal_time_constant=[.001, .2] s  thermal_time_constant_Cauer=[.001, .1, .2] s  thermal_time_constant_Foster=[7e-05, .0007, .01, .08] s  thermal_mass_initial_temperatures=[25, 25] degC  thermal_mass_initial_temperatures_Cauer=[25, 25, 25] degC  junction_thermal_mass=0.01 J/K  steadyState_Foster=simscape.enum.onoff.on  Tvec_initial_Foster=[25, 25, 25, 25] degC  junction_temperature_specify=off  junction_temperature_priority=None  junction_temperature=25 degC  junction_temperature_nominal_specify=off  junction_temperature_nominal_unit=degC  junction_temperature_nominal_value=1  vT_specify=off  vT_priority=None  vT=0 V  vT_nominal_specify=off  vT_nominal_unit=V  vT_nominal_value=1  Qj_specify=off  Qj_priority=None  Qj=0 W  Qj_nominal_specify=off  Qj_nominal_unit=W  Qj_nominal_value=1
      settings: SourceProductBaseCode=PS  LogSimulationData=on  InternalSimscapePortConfiguration="{\"Bottom\":[],\"Left\":[{\"id\":\"G\",\"label\":\"\",\"type\":\"input\"}],\"Right\":[{\"id\":\"A\",\"label\":\"\",\"type\":\"foundation.electrical.electrical\"},{\"id\":\"K\",\"label\":\"\",\"type\":\"foundation.electrical.electrical\"}],\"Top\":[]}"
  Thyristor 6 : ee_lib/Semiconductors & Converters/Thyristor (Piecewise Linear)  Vf=0.8 V  Ron=0.001 Ohm  Goff=1.0000e-05 1/Ohm  Vgt=6 V  Ih=0.01 A  diode_param=1  diode_Vf=0.8 V  diode_Ron=0.001 Ohm  diode_Goff=1e-5 1/Ohm  diode_C=5e-8 F  diode_iRM=-235 A  diode_iF=300 A  diode_idot=-50 A/us  diode_trr_param=1  diode_trr_factor=3  diode_trr=15 us  diode_Qrr=1.5e+3 s*uA  thermal_loss_option=ee.enum.converters.thermalLossOption.constantvalues  Von_data=[0, .1, .6, .8, 1, 1.3, 1.6, 2, 2.4; 0, .1, .7, 1, 1.2, 1.5, 1.9, 2.4, 2.8] V  Tj=[298.15, 398.15] K  Iout_data=[0, .1, 1, 5, 10, 20, 40, 70, 100] A  Eon_data=[0, .0024, .024, .12, .2, .48, 1.04, 2.16, 3.24; 0, .003, .03, .15, .25, .6, 1.3, 2.7, 4.05] * 1e-3 J  Tj_loss=[298.15, 398.15] K  Iout_data_loss=[0, .1, 1, 5, 10, 20, 40, 70, 100] A  Eon_scalar=22.86e-3 J  Eoff_natural_commutation=10e-3 J  Voff=300 V  Iout_scalar=600 A  onCurrentMeasDelay=1e-4 s  diodeModelType=ee.enum.converters.diodeModelType.pwl  diodeTableType=ee.enum.diode.tableType.IfMat  diode_IfMat=[.07, .12, .19, 1.75, 4.24, 7.32, 11.2; .16, .3, .72, 2.14, 4.02, 6.35, 9.12] A  diode_VfMat=[.9, 1.15, 1.25, 1.5, 1.75, 2.17, 2.6, 2.85; .58, .68, .75, 1.1, 1.38, 1.77, 2.27, 2.7] V  diode_TjVec=[25, 125] degC  diode_VfVec=[.5, .7, .9, 1.3, 1.7, 2.1, 2.5] V  diode_IfVec=[.1, .2, .5, 1, 2, 4, 7, 10] A  thermal_network_parameterization=ee.enum.thermalNetworkTopology.external  Rth=[.08, .5] K/W  Rth_Cauer=[.08, .1, .5] K/W  Rth_Foster=[.08, .14, .22, .16] K/W  thermal_mass_parameterization=ee.enum.thermalNetwork.timeconstant  thermal_mass=[.01, .5] J/K  thermal_mass_Cauer=[.01, .1, .5] J/K  thermal_mass_Foster=[.001, .005, .05, .5] J/K  thermal_time_constant=[.001, .2] s  thermal_time_constant_Cauer=[.001, .1, .2] s  thermal_time_constant_Foster=[7e-05, .0007, .01, .08] s  thermal_mass_initial_temperatures=[25, 25] degC  thermal_mass_initial_temperatures_Cauer=[25, 25, 25] degC  junction_thermal_mass=0.01 J/K  steadyState_Foster=simscape.enum.onoff.on  Tvec_initial_Foster=[25, 25, 25, 25] degC  junction_temperature_specify=off  junction_temperature_priority=None  junction_temperature=25 degC  junction_temperature_nominal_specify=off  junction_temperature_nominal_unit=degC  junction_temperature_nominal_value=1  vT_specify=off  vT_priority=None  vT=0 V  vT_nominal_specify=off  vT_nominal_unit=V  vT_nominal_value=1  Qj_specify=off  Qj_priority=None  Qj=0 W  Qj_nominal_specify=off  Qj_nominal_unit=W  Qj_nominal_value=1
      settings: SourceProductBaseCode=PS  InternalSimscapePortConfiguration="{\"Bottom\":[],\"Left\":[{\"id\":\"G\",\"label\":\"\",\"type\":\"input\"}],\"Right\":[{\"id\":\"A\",\"label\":\"\",\"type\":\"foundation.electrical.electrical\"},{\"id\":\"K\",\"label\":\"\",\"type\":\"foundation.electrical.electrical\"}],\"Top\":[]}"
  Thyristor{1..4} (4 alike) : ee_lib/Semiconductors & Converters/Thyristor (Piecewise Linear)  Vf=0.8 V  Ron=0.001 Ohm  Goff=1.0000e-05 1/Ohm  Vgt=6 V  Ih=0.01 A  diode_param=1  diode_Vf=0.8 V  diode_Ron=0.001 Ohm  diode_Goff=1e-5 1/Ohm  diode_C=5e-8 F  diode_iRM=-235 A  diode_iF=300 A  diode_idot=-50 A/us  diode_trr_param=1  diode_trr_factor=3  diode_trr=15 us  diode_Qrr=1.5e+3 s*uA  thermal_loss_option=ee.enum.converters.thermalLossOption.constantvalues  Von_data=[0, .1, .6, .8, 1, 1.3, 1.6, 2, 2.4; 0, .1, .7, 1, 1.2, 1.5, 1.9, 2.4, 2.8] V  Tj=[298.15, 398.15] K  Iout_data=[0, .1, 1, 5, 10, 20, 40, 70, 100] A  Eon_data=[0, .0024, .024, .12, .2, .48, 1.04, 2.16, 3.24; 0, .003, .03, .15, .25, .6, 1.3, 2.7, 4.05] * 1e-3 J  Tj_loss=[298.15, 398.15] K  Iout_data_loss=[0, .1, 1, 5, 10, 20, 40, 70, 100] A  Eon_scalar=22.86e-3 J  Eoff_natural_commutation=10e-3 J  Voff=300 V  Iout_scalar=600 A  onCurrentMeasDelay=1e-4 s  diodeModelType=ee.enum.converters.diodeModelType.pwl  diodeTableType=ee.enum.diode.tableType.IfMat  diode_IfMat=[.07, .12, .19, 1.75, 4.24, 7.32, 11.2; .16, .3, .72, 2.14, 4.02, 6.35, 9.12] A  diode_VfMat=[.9, 1.15, 1.25, 1.5, 1.75, 2.17, 2.6, 2.85; .58, .68, .75, 1.1, 1.38, 1.77, 2.27, 2.7] V  diode_TjVec=[25, 125] degC  diode_VfVec=[.5, .7, .9, 1.3, 1.7, 2.1, 2.5] V  diode_IfVec=[.1, .2, .5, 1, 2, 4, 7, 10] A  thermal_network_parameterization=ee.enum.thermalNetworkTopology.external  Rth=[.08, .5] K/W  Rth_Cauer=[.08, .1, .5] K/W  Rth_Foster=[.08, .14, .22, .16] K/W  thermal_mass_parameterization=ee.enum.thermalNetwork.timeconstant  thermal_mass=[.01, .5] J/K  thermal_mass_Cauer=[.01, .1, .5] J/K  thermal_mass_Foster=[.001, .005, .05, .5] J/K  thermal_time_constant=[.001, .2] s  thermal_time_constant_Cauer=[.001, .1, .2] s  thermal_time_constant_Foster=[7e-05, .0007, .01, .08] s  thermal_mass_initial_temperatures=[25, 25] degC  thermal_mass_initial_temperatures_Cauer=[25, 25, 25] degC  junction_thermal_mass=0.01 J/K  steadyState_Foster=simscape.enum.onoff.on  Tvec_initial_Foster=[25, 25, 25, 25] degC  junction_temperature_specify=off  junction_temperature_priority=None  junction_temperature=25 degC  junction_temperature_nominal_specify=off  junction_temperature_nominal_unit=degC  junction_temperature_nominal_value=1  vT_specify=off  vT_priority=None  vT=0 V  vT_nominal_specify=off  vT_nominal_unit=V  vT_nominal_value=1  Qj_specify=off  Qj_priority=None  Qj=0 W  Qj_nominal_specify=off  Qj_nominal_unit=W  Qj_nominal_value=1
      settings: SourceProductBaseCode=PS  InternalSimscapePortConfiguration="{\"Bottom\":[],\"Left\":[{\"id\":\"G\",\"label\":\"\",\"type\":\"input\"}],\"Right\":[{\"id\":\"A\",\"label\":\"\",\"type\":\"foundation.electrical.electrical\"},{\"id\":\"K\",\"label\":\"\",\"type\":\"foundation.electrical.electrical\"}],\"Top\":[]}"
  vA : fl_lib/Electrical/Electrical Sensors/Voltage Sensor
  vB : fl_lib/Electrical/Electrical Sensors/Voltage Sensor
  vC : fl_lib/Electrical/Electrical Sensors/Voltage Sensor
  a : PMIOPort  Side=Right
  b : PMIOPort  Port=2  Side=Right
  c : PMIOPort  Port=3  Side=Right
  A : PMIOPort  Port=4  Side=Left
  B : PMIOPort  Port=5  Side=Left
  C : PMIOPort  Port=6  Side=Left
  grd : PMIOPort  Port=7  Side=Right
  wires:
  firing curve/1 -> Firing Algorithm/1(firing curve)
  Relational Operator3/1 -> Data Type Conversion3/1
  Constant2/1 -> Relational Operator3/2, Relational Operator/2
  Clock/1 -> Relational Operator/1, Relational Operator3/1
  Data Type Conversion4/1 -> Simulink-PS Converter1/1
  Relational Operator/1 -> Data Type Conversion4/1
  Data Type Conversion3/1 -> Simulink-PS Converter2/1
  connections:
  Thyristor1/RConn2 -- vA/LConn1 -- A/RConn1 -- Thyristor 1/RConn1
  Firing Algorithm/LConn1 -- Thyristor 1/LConn1
  Thyristor 6/LConn1 -- Firing Algorithm/LConn6
  Thyristor 6/RConn2 -- vC/LConn1 -- C/RConn1 -- Thyristor4/RConn1
  Thyristor3/RConn2 -- vB/LConn1 -- B/RConn1 -- Thyristor2/RConn1
  Firing Algorithm/LConn2 -- Thyristor1/LConn1
  Thyristor4/LConn1 -- Firing Algorithm/LConn5
  Firing Algorithm/RConn1 -- vA/RConn1
  Thyristor3/LConn1 -- Firing Algorithm/LConn4
  vB/RConn1 -- Firing Algorithm/RConn2
  vC/RConn1 -- Firing Algorithm/RConn3
  Firing Algorithm/LConn3 -- Thyristor2/LConn1
  grd/RConn1 -- vC/RConn2 -- vB/RConn2 -- vA/RConn2
  Thyristor3/RConn1 -- Thyristor2/RConn2 -- b/RConn1 -- Circuit Breaker1/RConn1
  Thyristor 6/RConn1 -- Thyristor4/RConn2 -- Circuit Breaker2/RConn1 -- c/RConn1
  Electrical Reference/LConn1 -- Resistor/RConn1
  a/RConn1 -- Thyristor1/RConn1 -- Thyristor 1/RConn2 -- Circuit Breaker/RConn1
  Circuit Breaker/LConn2 -- Resistor/LConn1
  Circuit Breaker/LConn1 -- Circuit Breaker1/LConn1 -- Circuit Breaker2/LConn1 -- PS Subtract1/RConn1
  Simulink-PS Converter2/RConn1 -- Gain more than Vt1/LConn1
  PS Subtract1/LConn1 -- Gain more than Vt1/RConn1
  Gain less than Vt/LConn1 -- Simulink-PS Converter1/RConn1
  PS Subtract1/LConn2 -- Gain less than Vt/RConn1
  Circuit Breaker1/LConn2 -- Resistor3/LConn1
  Electrical Reference3/LConn1 -- Resistor3/RConn1
  Circuit Breaker2/LConn2 -- Resistor1/LConn1
  Electrical Reference1/LConn1 -- Resistor1/RConn1

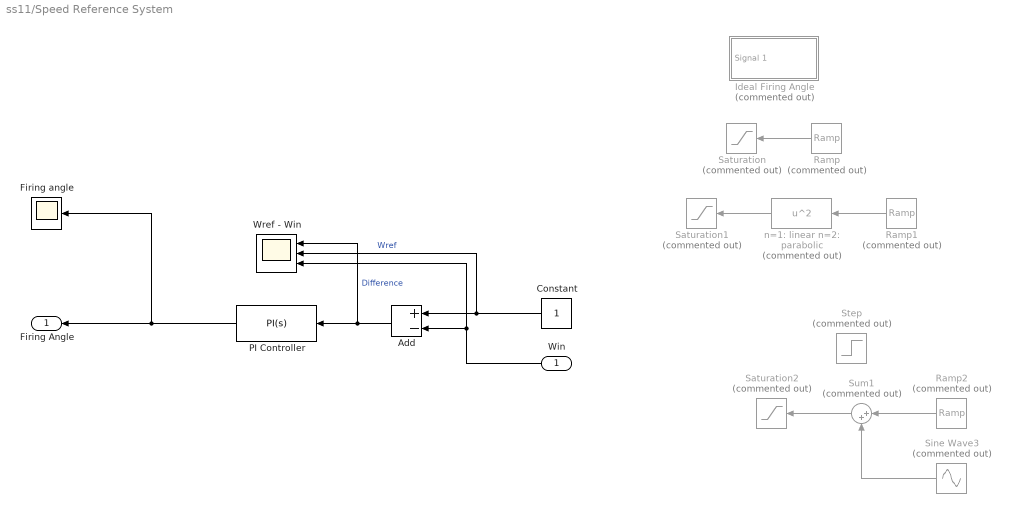
== system ss11/Speed Reference System ==
  Win : Inport
  Add : Sum  Inputs=+-
  Constant : Constant
  Firing angle : Scope
  Ideal Firing Angle : Subsystem  Tag=STV Subsys  Commented=on  LoadFcn=sigbuilder_block('load');  StartFcn=sigbuilder_block('start');  StopFcn=sigbuilder_block('stop');  ClipboardFcn=sigbuilder_block('clipboard');  mask(Sigbuilder block){tuvar=[0:10]}
      mask help: Simulink:masks:SigbuilderBlock_MD
      mask init:
      | if ~strcmp(get_param(bdroot(gcbh),'SimulationStatus'),'stopped') tuvar = sigbuilder_block('maskInit'); end
      settings: CopyFcn=sigbuilder_block('copy');  DeleteFcn=sigbuilder_block('delete');  ModelCloseFcn=sigbuilder_block('modelClose');  PreSaveFcn=sigbuilder_block('preSave');  PauseFcn=sigbuilder_block('pause');  ContinueFcn=sigbuilder_block('continue');  NameChangeFcn=sigbuilder_block('namechange');  OpenFcn=sigbuilder_block('open',[318 264.75 550.5 399.75 ]);  CloseFcn=sigbuilder_block('close');
      mask Display: plot(0, 0, 100, 100,[2, 2, 32, 32, 2], [68, 8, 8, 68, 68],[32, 2], [38, 38], [32, 19, 2],[53, 60, 44], [32, 17, 17, 2],[16, 16, 31, 31]);txt = getActiveGroup(gcbh);text(2, 100, txt,'verticalAlignment', 'top');
  PI Controller : slpidlib/PID Controller  Controller=PI  Form=Parallel  TimeDomain=Continuous-time  UseExternalTs=off  SampleTime=-1  IntegratorMethod=Forward Euler  FilterMethod=Forward Euler  ControllerParametersSource=internal  P=3  I=-6  D=0  UseFilter=on  N=100  TunerSelectOption=Frequency Response Based  ZeroCross=off  InitialConditionSource=internal  InitialConditionForIntegrator=2*pi/3  InitialConditionForFilter=0  DifferentiatorICPrevScaledInput=0  ExternalReset=none  TrackingMode=off  Kt=1  LimitOutput=on  SatLimitsSource=internal  UpperSaturationLimit=pi  LowerSaturationLimit=0  LinearizeAsGain=off  AntiWindupMode=back-calculation  Kb=1  RndMeth=Nearest  POutMin=[]  POutMax=[]  IOutMin=[]  IOutMax=[]  DOutMin=[]  DOutMax=[]  NOutMin=[]  NOutMax=[]  SumOutMin=[]  SumOutMax=[]  SaturationOutMin=[]  SaturationOutMax=[]  PParamMin=[]  PParamMax=[]  IParamMin=[]  IParamMax=[]  DParamMin=[]  DParamMax=[]  NParamMin=[]  NParamMax=[]  KbParamMin=[]  KbParamMax=[]  KtParamMin=[]  KtParamMax=[]  KbOutMin=[]  KbOutMax=[]  KtOutMin=[]  KtOutMax=[]  IntegratorOutMin=[]  IntegratorOutMax=[]  FilterOutMin=[]  FilterOutMax=[]  SumI1OutMin=[]  SumI1OutMax=[]  SumI2OutMin=[]  SumI2OutMax=[]  SumI3OutMin=[]  SumI3OutMax=[]  SumI4OutMin=[]  SumI4OutMax=[]  SumDOutMin=[]  SumDOutMax=[]  DifferentiatorOutMin=[]  DifferentiatorOutMax=[]  FilterDiffOutCoefMin=[]  FilterDiffOutCoefMax=[]  ReciprocalOutMin=[]  ReciprocalOutMax=[]  SumDenOutMin=[]  SumDenOutMax=[]  SumNumOutMin=[]  SumNumOutMax=[]  DivideOutMin=[]  DivideOutMax=[]  UdiffTsProdOutMin=[]  UdiffTsProdOutMax=[]  NTsProdOutMin=[]  NTsProdOutMax=[]  UintegralTsProdOutMin=[]  UintegralTsProdOutMax=[]  UngainTsProdOutMin=[]  UngainTsProdOutMax=[]  IntegratorContinuousStateAttributes=''  IntegratorStateMustResolveToSignalObject=off  IntegratorRTWStateStorageClass=Auto  FilterContinuousStateAttributes=''  FilterStateMustResolveToSignalObject=off  FilterRTWStateStorageClass=Auto  ParallelPVariant=InternalParameters  IdealPVariant=Disabled  IVariant=InternalParameters  DVariant=Disabled  IntegratorVariant=Continuous  SatVariant=Enabled  AWVariant=BackCalculation  PCopyVariant=Disabled  TRVariant=Disabled  FdbkBlocksVariant=Forward  IdealPFdbkVariant=Disabled  SatFdbkVariant=Disabled  DerivativeFilterVariant=Disabled  NVariant=Disabled  NCopyVariant=Disabled_SignalSpec  FilterICVariant=Disabled  IntegratorICVariant=InternalICs  ExternalResetVariant=Disabled  TRSumVariant=Passthrough  SumFdbkVariant=Disabled  SumVariant=Sum_PI  TsampFilterVariant=InternalTs  TsampNgainVariant=Passthrough  TsampIntegralVariant=Passthrough  ExternalSaturationOutDataTypeStr=Inherit: Same as second input
  Ramp : simulink/Sources/Ramp  Commented=on  slope=-5*pi/96  start=0  InitialOutput=5*pi/6
  Ramp1 : simulink/Sources/Ramp  Commented=on  slope=1/16  start=0  InitialOutput=0
  Ramp2 : simulink/Sources/Ramp  Commented=on  slope=-pi/16  start=0  InitialOutput=pi
  Saturation : Saturate  Commented=on  UpperLimit=pi  LowerLimit=0
  Saturation1 : Saturate  Commented=on  UpperLimit=1  LowerLimit=0  LinearizeAsGain=off  ZeroCross=off
  Saturation2 : Saturate  Commented=on  UpperLimit=10  LowerLimit=0
  Sine Wave3 : Sin  Commented=on  Amplitude=0.1  Frequency=2*pi/9  SampleTime=0
  Step : Step  Commented=on  Time=7.5  Before=0.5  SampleTime=0
  Sum1 : Sum  Commented=on  Inputs=|++
  Wref - Win : Scope  NumInputPorts=3
  n=1: linear n=2: parabolic : Fcn  Commented=on  Expr=u^2
  Firing Angle : Outport
  wires:
  n=1: linear n=2: parabolic/1 -> Saturation1/1
  Add/1 -> Wref - Win/1, PI Controller/1  "Difference"
  Constant/1 -> Wref - Win/2, Add/1  "Wref"
  Ramp1/1 -> n=1: linear n=2: parabolic/1
  Ramp/1 -> Saturation/1
  Win/1 -> Wref - Win/3, Add/2
  Sum1/1 -> Saturation2/1
  Sine Wave3/1 -> Sum1/2
  Ramp2/1 -> Sum1/1
  PI Controller/1 -> Firing angle/1, Firing Angle/1

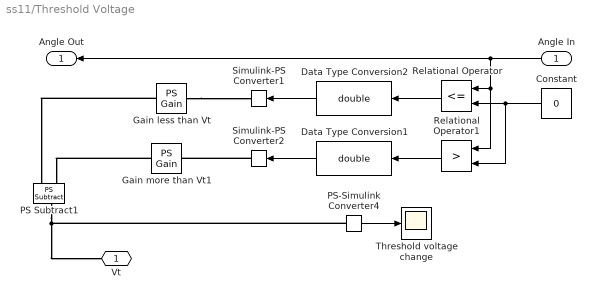
== system ss11/Threshold Voltage ==
  Angle In : Inport
  Constant : Constant  Value=0
  Data Type Conversion1 : DataTypeConversion  OutDataTypeStr=double
  Data Type Conversion2 : DataTypeConversion  OutDataTypeStr=double
  Gain less than Vt : fl_lib/Physical Signals/Functions/PS Gain  gain=-1 V
  Gain more than Vt1 : fl_lib/Physical Signals/Functions/PS Gain  gain=3 V
  PS Subtract1 : fl_lib/Physical Signals/Functions/PS Subtract
  PS-Simulink Converter4 : nesl_utility/PS-Simulink Converter  PhysicalDomain=network_engine_domain  SubClassName=ps_output  LeftPortType=input  RightPortType=output  PseudoPeriodic=off  Frequencies=[]  Unit=inherit  AffineConversion=off
      settings: SourceProductBaseCode=PW,SS
  Relational Operator : RelationalOperator  Operator=<=  OutDataTypeStr=boolean  RndMeth=Simplest
  Relational Operator1 : RelationalOperator  Operator=>  OutDataTypeStr=boolean  RndMeth=Simplest
  Simulink-PS Converter1 : nesl_utility/Simulink-PS Converter  PhysicalDomain=network_engine_domain  SubClassName=ps_input  LeftPortType=input  RightPortType=output  PseudoPeriodic=off  Frequencies=[]  NoiseDistribution=none  NoiseParameters=[]  Unit=1  AffineConversion=off  FilteringAndDerivatives=provide  SimscapeFilterOrder=1  InputFilterTimeConstant=0.001  UdotUserProvided=0
      settings: SourceProductBaseCode=PW,SS
  Simulink-PS Converter2 : nesl_utility/Simulink-PS Converter  PhysicalDomain=network_engine_domain  SubClassName=ps_input  LeftPortType=input  RightPortType=output  PseudoPeriodic=off  Frequencies=[]  NoiseDistribution=none  NoiseParameters=[]  Unit=1  AffineConversion=off  FilteringAndDerivatives=provide  SimscapeFilterOrder=1  InputFilterTimeConstant=0.001  UdotUserProvided=0
      settings: SourceProductBaseCode=PW,SS
  Threshold voltage change : Scope
  Vt : PMIOPort  Side=Right
  Angle Out : Outport
  wires:
  Data Type Conversion1/1 -> Simulink-PS Converter2/1
  Constant/1 -> Relational Operator1/2, Relational Operator/2
  Angle In/1 -> Angle Out/1, Relational Operator/1, Relational Operator1/1
  Relational Operator/1 -> Data Type Conversion2/1
  Data Type Conversion2/1 -> Simulink-PS Converter1/1
  PS-Simulink Converter4/1 -> Threshold voltage change/1
  Relational Operator1/1 -> Data Type Conversion1/1
  connections:
  Simulink-PS Converter2/RConn1 -- Gain more than Vt1/LConn1
  Gain less than Vt/LConn1 -- Simulink-PS Converter1/RConn1
  PS Subtract1/RConn1 -- PS-Simulink Converter4/LConn1 -- Vt/RConn1
  Gain more than Vt1/RConn1 -- PS Subtract1/LConn1
  Gain less than Vt/RConn1 -- PS Subtract1/LConn2
